simulink model "WhippleModel"  (Simulink 7.5)
settings: Solver=ode23s  StartTime=0.0  StopTime=stopTime  RelTol=1e-3
values from neighbouring files (symbols this model uses):
  A = zeros(mA + 2, nA + 2)    [system_state_space.m]
  B = zeros(mB + 2, nB)    [system_state_space.m]
  C = zeros(length(outputs), nA + 2)    [system_state_space.m]
  D = zeros(length(outputs), length(inputs))    [system_state_space.m]
  kDelta = guesses(1)    [generate_data.m]    (also in lookup_gains.m; system_state_space.m = gains(1))
  kPhi = guesses(3)    [generate_data.m]    (also in lookup_gains.m; system_state_space.m = gains(3))
  kPhiDot = guesses(2)    [generate_data.m]    (also in lookup_gains.m; system_state_space.m = gains(2))
  kPsi = guesses(4)    [generate_data.m]    (also in lookup_gains.m; system_state_space.m = gains(4))
  kY = guesses(5)    [generate_data.m]    (also in lookup_gains.m)
undefined symbols (not defined in the file or in its folder): closed, handlingFilterDen, handlingFilterNum, initialConditions, isFullSystem, isHandling, isPullPerturb, isRollInput, loopNumber, neuroDen, neuroNum, pathFilterDen, pathFilterNum, perturb, timeDelay
settings Model: Creator=moorepants  LastModifiedBy=moorepants
settings OptimizationCC: InlineParams=on  InlineInvariantSignals=on  InitFltsAndDblsToZero=on
settings DebuggingCC: SaveWithParameterizedLinksMsg=none  SignalResolutionControl=TryResolveAllWithWarning  MultiTaskDSMMsg=warning  MultiTaskCondExecSysMsg=none  StrictBusMsg=None
settings RTWCC: IncludeERTFirstTime=on
settings GRTTargetCC: TargetFcnLib=ansi_tfl_tmw.mat

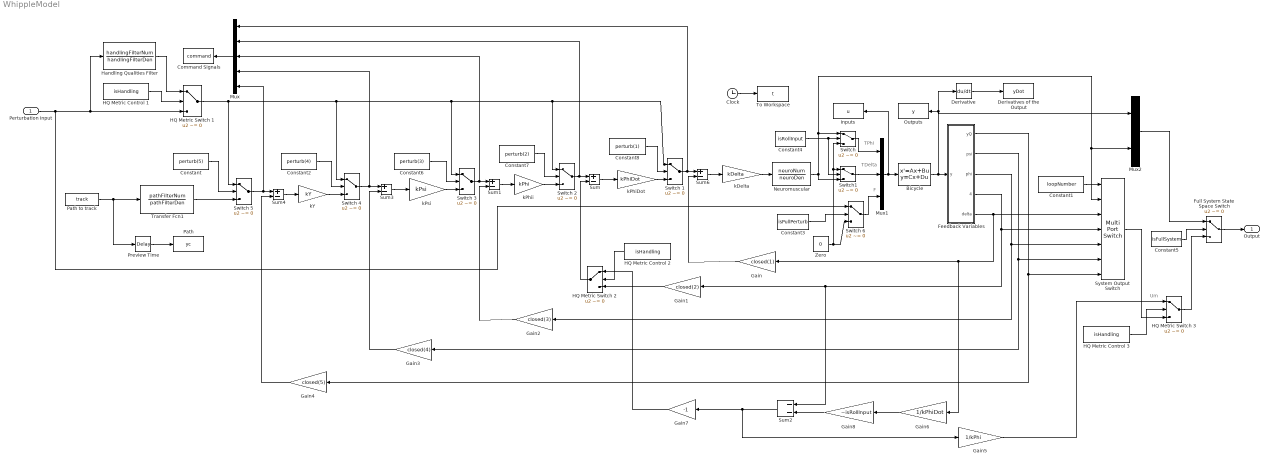
== system WhippleModel ==
  note: TPhi
  note: TDelta
  note: F
  note: Um
  Perturbation Input : Inport  OutDataType=fixdt(1, 16)  OutScaling=2^0
  Bicycle : StateSpace  A=A  B=B  C=C  D=D  X0=initialConditions
  Clock : Clock
      settings: Decimation=10
  Command Signals : ToWorkspace  VariableName=command  SampleTime=-1  SaveFormat=Array
  Constant : Constant  Value=perturb(5)  OutDataType=fixdt(1, 16)  OutScaling=2^0
  Constant1 : Constant  Value=loopNumber  OutDataType=fixdt(1, 16)  OutScaling=2^0
  Constant2 : Constant  Value=perturb(4)  OutDataType=fixdt(1, 16)  OutScaling=2^0
  Constant3 : Constant  Value=isPullPerturb  OutDataType=fixdt(1, 16)  OutScaling=2^0
  Constant4 : Constant  Value=isRollInput  OutDataType=fixdt(1, 16)  OutScaling=2^0
  Constant5 : Constant  Value=isFullSystem  OutDataType=fixdt(1, 16)  OutScaling=2^0
  Constant6 : Constant  Value=perturb(3)  OutDataType=fixdt(1, 16)  OutScaling=2^0
  Constant7 : Constant  Value=perturb(2)  OutDataType=fixdt(1, 16)  OutScaling=2^0
  Constant8 : Constant  Value=perturb(1)  OutDataType=fixdt(1, 16)  OutScaling=2^0
  Derivative : Derivative
  Derivatives of the Output : ToWorkspace  VariableName=yDot  SampleTime=-1  SaveFormat=Array
  Feedback Variables : Subsystem
  Full System State Space Switch : Switch  Criteria=u2 ~= 0  OutDataType=fixdt(1, 16)  OutScaling=2^0
  Gain : Gain  Gain=closed(1)  ParameterDataType=fixdt(1, 16)  ParameterScaling=2^0  OutDataType=fixdt(1, 16)  OutScaling=2^0
  Gain1 : Gain  Gain=closed(2)  ParameterDataType=fixdt(1, 16)  ParameterScaling=2^0  OutDataType=fixdt(1, 16)  OutScaling=2^0
  Gain2 : Gain  Gain=closed(3)  ParameterDataType=fixdt(1, 16)  ParameterScaling=2^0  OutDataType=fixdt(1, 16)  OutScaling=2^0
  Gain3 : Gain  Gain=closed(4)  ParameterDataType=fixdt(1, 16)  ParameterScaling=2^0  OutDataType=fixdt(1, 16)  OutScaling=2^0
  Gain4 : Gain  Gain=closed(5)  ParameterDataType=fixdt(1, 16)  ParameterScaling=2^0  OutDataType=fixdt(1, 16)  OutScaling=2^0
  Gain5 : Gain  Gain=1/kPhi  ParameterDataType=fixdt(1, 16)  ParameterScaling=2^0  OutDataType=fixdt(1, 16)  OutScaling=2^0
  Gain6 : Gain  Gain=1/kPhiDot  ParameterDataType=fixdt(1, 16)  ParameterScaling=2^0  OutDataType=fixdt(1, 16)  OutScaling=2^0
  Gain7 : Gain  Gain=-1  ParameterDataType=fixdt(1, 16)  ParameterScaling=2^0  OutDataType=fixdt(1, 16)  OutScaling=2^0
  Gain8 : Gain  Gain=~isRollInput  ParameterDataType=fixdt(1, 16)  ParameterScaling=2^0  OutDataType=fixdt(1, 16)  OutScaling=2^0
  HQ Metric Control 1 : Constant  Value=isHandling  OutDataType=fixdt(1, 16)  OutScaling=2^0
  HQ Metric Control 2 : Constant  Value=isHandling  OutDataType=fixdt(1, 16)  OutScaling=2^0
  HQ Metric Control 3 : Constant  Value=isHandling  OutDataType=fixdt(1, 16)  OutScaling=2^0
  HQ Metric Switch 1 : Switch  Criteria=u2 ~= 0  OutDataType=fixdt(1, 16)  OutScaling=2^0
  HQ Metric Switch 2 : Switch  Criteria=u2 ~= 0  OutDataType=fixdt(1, 16)  OutScaling=2^0
  HQ Metric Switch 3 : Switch  Criteria=u2 ~= 0  OutDataType=fixdt(1, 16)  OutScaling=2^0
  Handling Qualities Filter : TransferFcn  Numerator=handlingFilterNum  Denominator=handlingFilterDen
  Inputs : ToWorkspace  VariableName=u  SampleTime=-1  SaveFormat=Array
  Mux : Mux  Inputs=5
  Mux1 : Mux  Inputs=3
  Mux2 : Mux  Inputs=2
  Neuromuscular : TransferFcn  Numerator=neuroNum  Denominator=neuroDen
  Outputs : ToWorkspace  VariableName=y  SampleTime=-1  SaveFormat=Array
  Path : ToWorkspace  VariableName=yc  SampleTime=-1  SaveFormat=Array
  Path to track : FromWorkspace  VariableName=track  SampleTime=0
  Preview Time : TransportDelay  DelayTime=timeDelay
  Sum{,1,3..4,6} (5 alike) : Sum  Inputs=+-  OutDataType=sfix(16)  OutScaling=2^0
  Sum2 : Sum  Inputs=--  OutDataType=sfix(16)  OutScaling=2^0
  Switch : Switch  Criteria=u2 ~= 0  OutDataType=fixdt(1, 16)  OutScaling=2^0
  Switch {1..6} (6 alike) : Switch  Criteria=u2 ~= 0  OutDataType=fixdt(1, 16)  OutScaling=2^0
  Switch1 : Switch  Criteria=u2 ~= 0  OutDataType=fixdt(1, 16)  OutScaling=2^0
  System Output Switch : MultiPortSwitch  DataPortOrder=Zero-based contiguous  Inputs=6  zeroidx=on  OutDataType=fixdt(1, 16)  OutScaling=2^0
  To Workspace : ToWorkspace  VariableName=t  SampleTime=-1  SaveFormat=Array
  Transfer Fcn1 : TransferFcn  Numerator=pathFilterNum  Denominator=pathFilterDen
  Zero : Constant  Value=0  OutDataType=fixdt(1, 16)  OutScaling=2^0
  kDelta : Gain  Gain=kDelta  ParameterDataType=sfix(16)  ParameterScaling=2^0  OutDataType=sfix(16)  OutScaling=2^0
  kPhiDot : Gain  Gain=kPhiDot  ParameterDataType=sfix(16)  ParameterScaling=2^0  OutDataType=sfix(16)  OutScaling=2^0
  kPhii : Gain  Gain=kPhi  ParameterDataType=sfix(16)  ParameterScaling=2^0  OutDataType=sfix(16)  OutScaling=2^0
  kPsi : Gain  Gain=kPsi  ParameterDataType=sfix(16)  ParameterScaling=2^0  OutDataType=sfix(16)  OutScaling=2^0
  kY : Gain  Gain=kY  ParameterDataType=sfix(16)  ParameterScaling=2^0  OutDataType=sfix(16)  OutScaling=2^0
  Output : Outport  OutDataType=sfix(16)  OutScaling=2^0
  wires:
  Sum/1 -> kPhiDot/1
  Clock/1 -> To Workspace/1
  Mux1/1 -> Inputs/1, Bicycle/1
  Bicycle/1 -> Feedback Variables/1(y), Derivative/1, Outputs/1, Mux2/1
  Preview Time/1 -> Path/1
  Sum1/1 -> kPhii/1
  Sum3/1 -> kPsi/1
  Sum4/1 -> kY/1
  Constant1/1 -> System Output Switch/1
  Sum6/1 -> kDelta/1
  kDelta/1 -> Neuromuscular/1
  kPhiDot/1 -> Switch 1/3
  kPhii/1 -> Switch 2/3
  kPsi/1 -> Switch 3/3
  kY/1 -> Switch 4/3
  Switch 1/1 -> Sum6/1, Mux/1
  Switch 2/1 -> Sum/1, Mux/2
  Switch 3/1 -> Sum1/1, Mux/3
  Switch 4/1 -> Sum3/1, Mux/4
  Feedback Variables/5(delta) -> System Output Switch/3, Gain/1, Gain6/1
  Perturbation Input/1 -> HQ Metric Switch 1/3, Handling Qualities Filter/1, Switch 6/1
  Switch 5/1 -> Sum4/1, Mux/5
  Feedback Variables/1(yQ) -> Gain4/1, System Output Switch/7
  Gain/1 -> Sum6/2
  Gain3/1 -> Sum3/2
  Gain2/1 -> Sum1/2
  Feedback Variables/3(phi) -> System Output Switch/5, Gain2/1
  Feedback Variables/2(psi) -> Gain3/1, System Output Switch/6
  Feedback Variables/4(phiDot) -> System Output Switch/4, Gain1/1, Sum2/1
  Gain4/1 -> Sum4/2
  Mux/1 -> Command Signals/1
  HQ Metric Switch 1/1 -> Switch 1/1, Switch 2/1, Switch 3/1, Switch 4/1, Switch 5/1
  Sum2/1 -> Gain7/1, Gain5/1
  HQ Metric Switch 2/1 -> Sum/2
  Gain1/1 -> HQ Metric Switch 2/3
  Gain7/1 -> HQ Metric Switch 2/1
  Handling Qualities Filter/1 -> HQ Metric Switch 1/1
  HQ Metric Control 1/1 -> HQ Metric Switch 1/2
  HQ Metric Control 2/1 -> HQ Metric Switch 2/2
  Gain5/1 -> HQ Metric Switch 3/1
  System Output Switch/1 -> HQ Metric Switch 3/3
  HQ Metric Control 3/1 -> HQ Metric Switch 3/2
  Transfer Fcn1/1 -> Switch 5/3
  Constant/1 -> Switch 5/2
  Constant2/1 -> Switch 4/2
  Constant6/1 -> Switch 3/2
  Constant7/1 -> Switch 2/2
  Switch1/1 -> Mux1/2
  Switch/1 -> Mux1/1
  Constant4/1 -> Switch/2, Switch1/2
  Neuromuscular/1 -> Switch1/3, Switch/1, System Output Switch/2, Mux2/2
  Constant8/1 -> Switch 1/2
  Gain6/1 -> Gain8/1
  Gain8/1 -> Sum2/2
  Derivative/1 -> Derivatives of the Output/1
  Path to track/1 -> Transfer Fcn1/1, Preview Time/1
  Switch 6/1 -> Mux1/3
  Constant3/1 -> Switch 6/2
  Zero/1 -> Switch 6/3, Switch/3, Switch1/1
  Constant5/1 -> Full System State Space Switch/2
  HQ Metric Switch 3/1 -> Full System State Space Switch/3
  Full System State Space Switch/1 -> Output/1
  Mux2/1 -> Full System State Space Switch/1

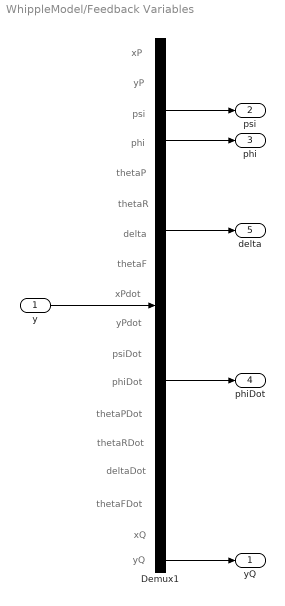
== system WhippleModel/Feedback Variables ==
  note: xP
  note: yP
  note: psi
  note: phi
  note: thetaP
  note: thetaR
  note: delta
  note: thetaF
  note: xPdot
  note: yPdot
  note: psiDot
  note: phiDot
  note: thetaPDot
  note: thetaRDot
  note: deltaDot
  note: thetaFDot
  note: xQ
  note: yQ
  y : Inport  OutDataType=fixdt(1, 16)  OutScaling=2^0
  Demux1 : Demux  Outputs=18
  yQ : Outport  OutDataType=fixdt(1, 16)  OutScaling=2^0
  psi : Outport  Port=2  OutDataType=fixdt(1, 16)  OutScaling=2^0
  phi : Outport  Port=3  OutDataType=fixdt(1, 16)  OutScaling=2^0
  phiDot : Outport  Port=4  OutDataType=fixdt(1, 16)  OutScaling=2^0
  delta : Outport  Port=5  OutDataType=fixdt(1, 16)  OutScaling=2^0
  wires:
  y/1 -> Demux1/1
  Demux1/3 -> psi/1
  Demux1/4 -> phi/1
  Demux1/7 -> delta/1
  Demux1/12 -> phiDot/1
  Demux1/18 -> yQ/1
